simulink model "simulink_model"  (R2024a)
settings: Solver=VariableStepAuto  StartTime=0.0  StopTime=10.0  RelTol=1e-3
values from neighbouring files (symbols this model uses):
  A = [-1.064 1.000; 290.26 0.00]    [model.m]
  B = [-0.25; -331.40]    [model.m]
  C = [-123.34 0.00; 0.00 1.00]    [model.m]
  D = [-13.51; 0.00]    [model.m]
  dT1 = 0.75    [model.m]
  dT2 = 0.25    [model.m]
  ELEV_INIT = 10000    [model.m]
  LAT_INIT = 34.2329    [model.m]
  LON_INIT = -119.4573    [model.m]
  Vel = 1021.08    [model.m]
undefined symbols (not defined in the file or in its folder): Earth, K, L, WGS84
libraries: simulink x2, slpidlib x1, aerolibtransform2 x1
settings Model: Creator=NathanIgot  LastModifiedBy=ennde
settings RTWCC: GPUComputeCapability=3.5

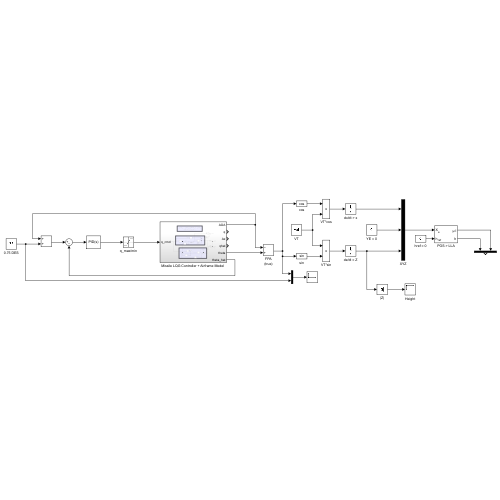
[thumbnail: Simulink's stored preview of the top-level diagram]
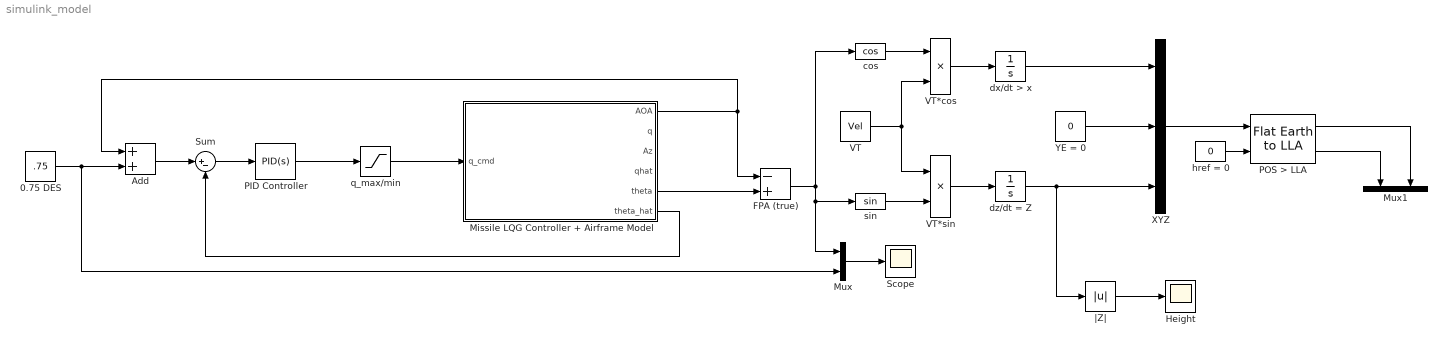
== system simulink_model ==
  0.75 DES : Constant  Value=.75
  Add : Sum
  FPA (true) : Sum  Inputs=-+
  Height : Scope
  "Missile LQG Controller + Airframe Model " : Subsystem
  Mux : Mux  Inputs=2
  Mux1 : Mux  Inputs=2
  PID Controller : slpidlib/PID Controller  Controller=PID  Form=Parallel  TimeDomain=Continuous-time  UseExternalTs=off  SampleTime=-1  IntegratorMethod=Forward Euler  FilterMethod=Forward Euler  ControllerParametersSource=internal  P=-1  I=0  UseKiTs=off  D=0  UseExternalDerivativeSource=off  N=100  UseFilter=on  TunerSelectOption=Transfer Function Based (PID Tuner App)  InitialConditionSource=internal  InitialConditionForIntegrator=0  InitialConditionForFilter=0  DifferentiatorICPrevScaledInput=0  ExternalReset=none  TrackingMode=off  Kt=1  LimitOutput=off  SatLimitsSource=internal  UpperSaturationLimit=inf  LowerSaturationLimit=-inf  LinearizeAsGain=on  AntiWindupMode=none  Kb=1  LimitIntegrator=off  UpperIntegratorSaturationLimit=inf  LowerIntegratorSaturationLimit=-inf  POutMin=[]  POutMax=[]  IOutMin=[]  IOutMax=[]  DOutMin=[]  DOutMax=[]  NOutMin=[]  NOutMax=[]  SumOutMin=[]  SumOutMax=[]  SaturationOutMin=[]  SaturationOutMax=[]  PParamMin=[]  PParamMax=[]  IParamMin=[]  IParamMax=[]  DParamMin=[]  DParamMax=[]  NParamMin=[]  NParamMax=[]  KbParamMin=[]  KbParamMax=[]  KtParamMin=[]  KtParamMax=[]  KbOutMin=[]  KbOutMax=[]  KtOutMin=[]  KtOutMax=[]  IntegratorOutMin=[]  IntegratorOutMax=[]  FilterOutMin=[]  FilterOutMax=[]  SumI1OutMin=[]  SumI1OutMax=[]  SumI2OutMin=[]  SumI2OutMax=[]  SumI3OutMin=[]  SumI3OutMax=[]  SumI4OutMin=[]  SumI4OutMax=[]  SumDOutMin=[]  SumDOutMax=[]  DifferentiatorOutMin=[]  DifferentiatorOutMax=[]  FilterDiffOutCoefMin=[]  FilterDiffOutCoefMax=[]  ReciprocalOutMin=[]  ReciprocalOutMax=[]  SumDenOutMin=[]  SumDenOutMax=[]  SumNumOutMin=[]  SumNumOutMax=[]  DivideOutMin=[]  DivideOutMax=[]  UdiffTsProdOutMin=[]  UdiffTsProdOutMax=[]  NTsProdOutMin=[]  NTsProdOutMax=[]  UintegralTsProdOutMin=[]  UintegralTsProdOutMax=[]  UngainTsProdOutMin=[]  UngainTsProdOutMax=[]  ClampingZeroOutDataTypeStr=Inherit: Inherit via back propagation  ClampingZeroOutMin=[]  ClampingZeroOutMax=[]  FilterDenConstantOutDataTypeStr=Inherit: Inherit via back propagation  FilterDenConstantOutMin=[]  FilterDenConstantOutMax=[]  PCopyOutDataTypeStr=Inherit: Inherit via back propagation  PCopyOutMin=[]  PCopyOutMax=[]  NCopyOutDataTypeStr=Inherit: Inherit via back propagation  NCopyOutMin=[]  NCopyOutMax=[]  IntegratorContinuousStateAttributes=''  IntegratorStateMustResolveToSignalObject=off  IntegratorRTWStateStorageClass=Auto  FilterContinuousStateAttributes=''  FilterStateMustResolveToSignalObject=off  FilterRTWStateStorageClass=Auto  ParallelPVariant=InternalParameters  IdealPVariant=Disabled  IVariant=InternalParameters  DVariant=InternalParameters  IntegratorVariant=Continuous  SatVariant=Disabled  AWVariant=Passthrough  PCopyVariant=Disabled  TRVariant=Disabled  FdbkBlocksVariant=Forward  IdealPFdbkVariant=Disabled  SatFdbkVariant=Disabled  DerivativeFilterVariant=ContFilter  NVariant=InternalParameters  NCopyVariant=Disabled  FilterICVariant=InternalICsFilter  IntegratorICVariant=InternalICs  ExternalResetVariant=Disabled  TRSumVariant=Passthrough  SumFdbkVariant=Disabled  SumVariant=Sum_PID  TsampFilterVariant=InternalTs  TsampNgainVariant=Passthrough  TsampIntegralVariant=Passthrough  ExternalSaturationOutDataTypeStr=Inherit: Same as second input  DerivativeSourceVariant=ErrorSignal
  POS > LLA : aerolibtransform2/Flat Earth to LLA  units=Metric (MKS)  ptype=Earth (WGS84)  F=1/298.257223563  R=6378137  refPosPort=off  LL0=[LAT_INIT LON_INIT]  psi=yaw_init
  Scope : Scope
  Sum : Sum  Inputs=|+-
  VT : Constant  Value=Vel
  VT*cos : Product
  VT*sin : Product
  XYZ : Mux  Inputs=3
  YE = 0 : Constant  Value=0
  cos : Trigonometry  Operator=cos
  dx/dt > x : Integrator
  dz/dt = Z : Integrator  InitialCondition=-ELEV_INIT
  href = 0 : Constant  Value=0
  q_max/min : Saturate
  sin : Trigonometry
  |Z| : Abs  SaturateOnIntegerOverflow=off
  wires:
  PID Controller/1 -> q_max/min/1
  q_max/min/1 -> "Missile LQG Controller + Airframe Model "/1(q_cmd)
  Sum/1 -> PID Controller/1
  "Missile LQG Controller + Airframe Model "/6(theta_hat) -> Sum/2
  Add/1 -> Sum/1
  "Missile LQG Controller + Airframe Model "/1(AOA) -> FPA (true)/1, Add/1
  0.75 DES/1 -> Mux/2, Add/2
  FPA (true)/1 -> cos/1, Mux/1, sin/1
  "Missile LQG Controller + Airframe Model "/5(theta) -> FPA (true)/2
  Mux/1 -> Scope/1
  sin/1 -> VT*sin/2
  cos/1 -> VT*cos/1
  VT/1 -> VT*cos/2, VT*sin/1
  VT*cos/1 -> dx/dt > x/1
  VT*sin/1 -> dz/dt = Z/1
  dx/dt > x/1 -> XYZ/1
  YE = 0/1 -> XYZ/2
  dz/dt = Z/1 -> |Z|/1, XYZ/3
  |Z|/1 -> Height/1
  XYZ/1 -> POS > LLA/1
  href = 0/1 -> POS > LLA/2
  POS > LLA/1 -> Mux1/2
  POS > LLA/2 -> Mux1/1

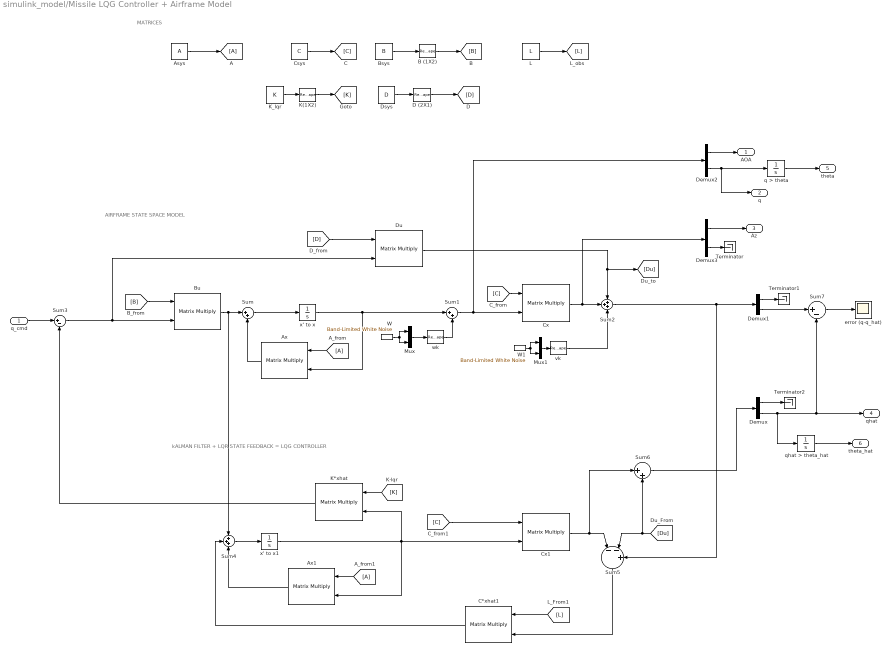
== system simulink_model/Missile LQG Controller + Airframe Model  ==
  note: kALMAN FILTER + LQR STATE FEEDBACK = LQG CONTROLLER
  note: AIRFRAME STATE SPACE MODEL
  note: MATRICES
  q_cmd : Inport
  A : Goto
  A_from : From
  A_from1 : From
  Asys : Constant  Value=A
  Ax : Product  Multiplication=Matrix(*)
  Ax1 : Product  Multiplication=Matrix(*)
  B (1X2) : Reshape  OutputDimensionality=Customize  OutputDimensions=[2,1]
  Bsys : Constant  Value=B
  Bu : Product  Multiplication=Matrix(*)
  C*xhat1 : Product  Multiplication=Matrix(*)
  Csys : Constant  Value=C
  Cx : Product  Multiplication=Matrix(*)
  Cx1 : Product  Multiplication=Matrix(*)
  D (2X1) : Reshape  OutputDimensionality=Customize  OutputDimensions=[2,1]
  Demux{,1..3} (4 alike) : Demux  Outputs=2
  Dsys : Constant  Value=D
  Du : Product  Multiplication=Matrix(*)
  K(1X2) : Reshape  OutputDimensionality=Customize  OutputDimensions=[1,2]
  K*xhat : Product  Multiplication=Matrix(*)
  K_lqr : Constant  Value=K
  L : Constant  Value=L
  Mux : Mux  Inputs=2
  Mux1 : Mux  Inputs=2
  Sum : Sum  Inputs=|++
  Sum1 : Sum  Inputs=|++
  Sum2 : Sum  Inputs=+++
  Sum3 : Sum  Inputs=|+-
  Sum4 : Sum  Inputs=+++
  Sum5 : Sum  Inputs=|--+
  Sum6 : Sum  Inputs=|++
  Sum7 : Sum  Inputs=|+-
  Terminator : Terminator
  Terminator1 : Terminator
  Terminator2 : Terminator
  W : simulink/Sources/Band-Limited White Noise  Cov=[0.00000001]  Ts=dT1  seed=[23341]
  W1 : simulink/Sources/Band-Limited White Noise  Cov=[0.00001]  Ts=dT2  seed=[23341]
  error (q-q_hat) : Scope
  q > theta : Integrator
  qhat > theta_hat : Integrator
  vk : Reshape  OutputDimensionality=Customize  OutputDimensions=[2,1]
  wk : Reshape  OutputDimensionality=Customize  OutputDimensions=[2,1]
  x' to x : Integrator
  x' to x1 : Integrator
  AOA : Outport
  q : Outport  Port=2
  Az : Outport  Port=3
  qhat : Outport  Port=4
  theta : Outport  Port=5
  theta_hat : Outport  Port=6
  wires:
  Sum/1 -> x' to x/1
  Demux3/2 -> Terminator/1
  x' to x/1 -> Sum1/1, Ax/2
  Cx1/1 -> Sum6/1, Sum5/1
  [L] -> C*xhat1/1
  Demux1/1 -> Terminator1/1
  Asys/1 -> A/1
  [C] -> Cx/1
  Demux/2 -> qhat > theta_hat/1, qhat/1, Sum7/2
  Mux/1 -> wk/1
  [B] -> Bu/1
  Ax/1 -> Sum/2
  wk/1 -> Sum1/2
  Sum4/1 -> x' to x1/1
  Sum1/1 -> Cx/2, Demux2/1
  q_cmd/1 -> Sum3/1
  L/1 -> [L]
  qhat > theta_hat/1 -> theta_hat/1
  Dsys/1 -> D (2X1)/1
  Sum3/1 -> Du/2, Bu/2
  [Du] -> Sum5/2, Sum6/2
  Bsys/1 -> B (1X2)/1
  W1/1 -> Mux1/1, Mux1/2
  K_lqr/1 -> K(1X2)/1
  Mux1/1 -> vk/1
  [K] -> K*xhat/1
  W/1 -> Mux/1, Mux/2
  Sum6/1 -> Demux/1
  Du/1 -> [Du], Sum2/1
  Ax1/1 -> Sum4/3
  Bu/1 -> Sum/1, Sum4/1
  [D] -> Du/1
  Sum5/1 -> C*xhat1/2
  Cx/1 -> Demux3/1, Sum2/2
  K*xhat/1 -> Sum3/2
  K(1X2)/1 -> [K]
  Sum2/1 -> Sum5/3, Demux1/1
  C*xhat1/1 -> Sum4/2
  x' to x1/1 -> Ax1/2, K*xhat/2, Cx1/2
  Sum7/1 -> error (q-q_hat)/1
  vk/1 -> Sum2/3
  Demux2/2 -> q/1, q > theta/1
  A_from1/1 -> Ax1/1
  Csys/1 -> [C]
  A_from/1 -> Ax/1
  [C] -> Cx1/1
  Demux3/1 -> Az/1
  Demux1/2 -> Sum7/1
  q > theta/1 -> theta/1
  Demux2/1 -> AOA/1
  D (2X1)/1 -> [D]
  Demux/1 -> Terminator2/1
  B (1X2)/1 -> [B]
